simulink library "NeuroModelerLibrary"  (Simulink 10.2)
settings: Solver=ode45  StartTime=0.0  StopTime=10.0  RelTol=1e-3
libraries: $bdroot x672, simulink x5, neural x2
(part 3 of 5)

== system NeuroModelerLibrary/Simple Cells/Large PresynInh  NewNeuron v0.1 ==
  In1 : Inport
  In2 : Inport  Port=2
  In3 : Inport  Port=3
  In4 : Inport  Port=4
  In5 : Inport  Port=5
  C1 : Constant  Value=100
  C2 : Constant  Value=100
  Gain1 : Gain  Gain=0.5  OutDataTypeStr=Inherit: Same as input  ParamDataTypeStr=Inherit: Same as input
  Gain2 : Gain  Gain=-1  OutDataTypeStr=Inherit: Same as input  ParamDataTypeStr=Inherit: Same as input
  Gain3 : Gain  Gain=0.5  OutDataTypeStr=Inherit: Same as input  ParamDataTypeStr=Inherit: Same as input
  Gain4 : Gain  Gain=0.5  OutDataTypeStr=Inherit: Same as input  ParamDataTypeStr=Inherit: Same as input
  LTZone v0.1 : $bdroot/Neuron Elements/LTZone v0.1  Rc=1  Cc=0.001  RR=1  IT=0.005  T=10
  Neuro Membrane{,1..5} (6 alike) : $bdroot/Neuron Elements/Neuro Membrane v0.1  ACm=0.1  ARm=1  ECm=0.1  ERm=1
  Sum2 : Sum  InputSameDT=on  SaturateOnIntegerOverflow=on  OutDataTypeStr=Inherit: Same as first input
  Sum3 : Sum  InputSameDT=on  SaturateOnIntegerOverflow=on  OutDataTypeStr=Inherit: Same as first input
  Sum7 : Sum  Inputs=++++  InputSameDT=on  SaturateOnIntegerOverflow=on  OutDataTypeStr=Inherit: Same as first input
  Synapse PresynInh v0.1 - {1..3,5} (4 alike) : $bdroot/Neuron Elements/Synapse v0.1  SecretionTC=0.001  DecompositionTC=0.1  ksi=2  gamma=1
  Synapse PresynInh v0.1 -4 : $bdroot/Neuron Elements/Synapse v0.1  SecretionTC=0.001  DecompositionTC=0.1  ksi=2  gamma=1
  Out1 : Outport  VectorParamsAs1DForOutWhenUnconnected=off
  Out2 : Outport  Port=2  VectorParamsAs1DForOutWhenUnconnected=off
  Out3 : Outport  Port=3  VectorParamsAs1DForOutWhenUnconnected=off
  wires:
  In5/1 -> Synapse PresynInh v0.1 - 5/1
  Synapse PresynInh v0.1 - 5/1 -> Neuro Membrane5/1
  In4/1 -> Synapse PresynInh v0.1 -4/1
  Synapse PresynInh v0.1 -4/1 -> Neuro Membrane2/1
  In3/1 -> Synapse PresynInh v0.1 - 3/1
  Synapse PresynInh v0.1 - 3/1 -> Neuro Membrane3/1
  Synapse PresynInh v0.1 - 2/1 -> Neuro Membrane/1
  In2/1 -> Synapse PresynInh v0.1 - 2/1
  C2/1 -> Neuro Membrane1/2, Neuro Membrane4/2, Neuro Membrane5/2, Gain2/1
  Gain2/1 -> Neuro Membrane1/4, Neuro Membrane4/4, Neuro Membrane5/4
  Neuro Membrane2/2 -> Sum7/2
  Sum7/1 -> Gain1/1
  Neuro Membrane2/1 -> Sum7/1
  C1/1 -> LTZone v0.1/2
  In1/1 -> Synapse PresynInh v0.1 - 1/1
  Synapse PresynInh v0.1 - 1/1 -> Neuro Membrane1/1
  LTZone v0.1/1 -> Neuro Membrane4/3, Out2/1, Neuro Membrane2/3
  Neuro Membrane1/1 -> Neuro Membrane/2
  Neuro Membrane1/2 -> Neuro Membrane/4
  Neuro Membrane3/1 -> Neuro Membrane2/2
  Neuro Membrane3/2 -> Neuro Membrane2/4
  Neuro Membrane/1 -> Sum2/1
  Neuro Membrane/2 -> Sum3/1
  Sum3/1 -> Gain3/1
  Sum2/1 -> Gain4/1
  Neuro Membrane5/1 -> Sum2/2
  Neuro Membrane5/2 -> Sum3/2
  Gain1/1 -> LTZone v0.1/1
  LTZone v0.1/3 -> Out1/1
  Gain3/1 -> Neuro Membrane3/4
  Gain4/1 -> Neuro Membrane3/2
  Neuro Membrane4/1 -> Sum7/3
  Neuro Membrane4/2 -> Sum7/4
  LTZone v0.1/2 -> Out3/1

== system NeuroModelerLibrary/Simple Cells/Simple Cell ==
  Stimulate : Inport
  Arresting : Inport  Port=2
  C1 : Constant
  C2 : Constant
  C3 : Constant  Value=-1
  LTZone : $bdroot/Neuron Elements/LTZone  NM=1  FB=1.7  IT=0.005  T=0.001
  Simple Membrane : $bdroot/Neuron Elements/Simple Membrane  ACm=1e-9  ARm=1e7  ECm=1e-9  ERm=1e7  ARFm=1e8  ERFm=1e8
  Sum7 : Sum  InputSameDT=on  SaturateOnIntegerOverflow=on  OutDataTypeStr=Inherit: Same as first input
  Synapse : $bdroot/Neuron Elements/Synapse  SecretionTC=0.001  DecompositionTC=0.01  UseKsi=on  ksi=2  gamma=1e8
  Synapse1 : $bdroot/Neuron Elements/Synapse  SecretionTC=0.001  DecompositionTC=0.01  UseKsi=on  ksi=2  gamma=1e8
  Out : Outport  VectorParamsAs1DForOutWhenUnconnected=off
  Visual : Outport  Port=2  VectorParamsAs1DForOutWhenUnconnected=off
  Potential : Outport  Port=3  VectorParamsAs1DForOutWhenUnconnected=off
  wires:
  LTZone/2 -> Visual/1
  LTZone/3 -> Out/1
  C1/1 -> LTZone/2
  Stimulate/1 -> Synapse/1
  Arresting/1 -> Synapse1/1
  Sum7/1 -> LTZone/1, Potential/1
  LTZone/1 -> Simple Membrane/3
  C2/1 -> Simple Membrane/2
  C3/1 -> Simple Membrane/4
  Simple Membrane/1 -> Sum7/1
  Simple Membrane/2 -> Sum7/2
  Synapse/1 -> Simple Membrane/1
  Synapse1/1 -> Simple Membrane/5

== system NeuroModelerLibrary/Simple Cells/Simple Cell - Inertial ==
  Stimulate : Inport
  Arresting : Inport  Port=2
  C1 : Constant
  C2 : Constant
  C3 : Constant  Value=-1
  LTZone : $bdroot/Neuron Elements/LTZone  NM=1  FB=1.7  IT=0.005  T=0.00001
  Simple Membrane : $bdroot/Neuron Elements/Simple Membrane  ACm=1e-9  ARm=1e7  ECm=1e-9  ERm=1e7  ARFm=1e8  ERFm=1e8
  Simple Membrane1 : $bdroot/Neuron Elements/Simple Membrane  ACm=1e-7  ARm=1e7  ECm=1e-7  ERm=1e7  ARFm=1e8  ERFm=1e8
  Sum1 : Sum  InputSameDT=on  SaturateOnIntegerOverflow=on  OutDataTypeStr=Inherit: Same as first input
  Sum7 : Sum  InputSameDT=on  SaturateOnIntegerOverflow=on  OutDataTypeStr=Inherit: Same as first input
  Synapse : Subsystem  AncestorBlock=NeuroModelerLibrary/Neuron Elements/Synapse  mask{SecretionTC=0.001, DecompositionTC=0.01, ksi=2, gamma=1e8}
      mask prompts: SecretionTC "Mediator Secretion"; DecompositionTC "Mediator Decomposition"
  Synapse1 : Subsystem  AncestorBlock=NeuroModelerLibrary/Neuron Elements/Synapse  mask{SecretionTC=0.001, DecompositionTC=0.01, ksi=2, gamma=1e8}
      mask prompts: SecretionTC "Mediator Secretion"; DecompositionTC "Mediator Decomposition"
  Out : Outport  VectorParamsAs1DForOutWhenUnconnected=off
  Visual : Outport  Port=2  VectorParamsAs1DForOutWhenUnconnected=off
  Potential : Outport  Port=3  VectorParamsAs1DForOutWhenUnconnected=off
  wires:
  Synapse1/1(Out1) -> Simple Membrane/5
  Synapse/1(Out1) -> Simple Membrane/1
  C3/1 -> Simple Membrane/4
  C2/1 -> Simple Membrane/2
  Sum7/1 -> LTZone/1
  Arresting/1 -> Synapse1/1(In1)
  Stimulate/1 -> Synapse/1(In1)
  C1/1 -> LTZone/2
  LTZone/3 -> Out/1
  LTZone/2 -> Visual/1
  Simple Membrane/1 -> Simple Membrane1/2, Sum1/1
  Simple Membrane/2 -> Simple Membrane1/4, Sum1/2
  Simple Membrane1/1 -> Sum7/1
  Simple Membrane1/2 -> Sum7/2
  LTZone/1 -> Simple Membrane1/3
  Sum1/1 -> Potential/1

== system NeuroModelerLibrary/Simple Cells/Simple Cell MembraneCap ==
  Stimulate : Inport
  Arresting : Inport  Port=2
  C1 : Constant
  C2 : Constant
  C3 : Constant  Value=-1
  LTZone : $bdroot/Neuron Elements/LTZone  NM=1  FB=1.7  IT=0.005  T=0.00001
  Simple Membrane : $bdroot/Neuron Elements/Simple Membrane  ACm=1e-9  ARm=1e7  ECm=1e-9  ERm=1e7  ARFm=1e8  ERFm=1e8
  Simple Membrane1 : $bdroot/Neuron Elements/Simple Membrane  ACm=1e-7  ARm=1e7  ECm=1e-7  ERm=1e7  ARFm=1e8  ERFm=1e8
  Sum1 : Sum  InputSameDT=on  SaturateOnIntegerOverflow=on  OutDataTypeStr=Inherit: Same as first input
  Sum7 : Sum  InputSameDT=on  SaturateOnIntegerOverflow=on  OutDataTypeStr=Inherit: Same as first input
  Synapse : Subsystem  AncestorBlock=NeuroModelerLibrary/Neuron Elements/Synapse  mask{SecretionTC=0.001, DecompositionTC=0.01, ksi=2, gamma=1e8}
      mask prompts: SecretionTC "Mediator Secretion"; DecompositionTC "Mediator Decomposition"
  Synapse1 : Subsystem  AncestorBlock=NeuroModelerLibrary/Neuron Elements/Synapse  mask{SecretionTC=0.001, DecompositionTC=0.01, ksi=2, gamma=1e8}
      mask prompts: SecretionTC "Mediator Secretion"; DecompositionTC "Mediator Decomposition"
  Out : Outport
  Visual : Outport  Port=2
  Potential : Outport  Port=3
  wires:
  Sum1/1 -> Potential/1
  LTZone/1 -> Simple Membrane1/3
  Simple Membrane1/2 -> Sum7/2
  Simple Membrane1/1 -> Sum7/1
  Simple Membrane/2 -> Sum1/2, Simple Membrane1/4
  Simple Membrane/1 -> Sum1/1, Simple Membrane1/2
  LTZone/2 -> Visual/1
  LTZone/3 -> Out/1
  C1/1 -> LTZone/2
  Stimulate/1 -> Synapse/1(In1)
  Arresting/1 -> Synapse1/1(In1)
  Sum7/1 -> LTZone/1
  C2/1 -> Simple Membrane/2
  C3/1 -> Simple Membrane/4
  Synapse/1(Out1) -> Simple Membrane/1
  Synapse1/1(Out1) -> Simple Membrane/5

== system NeuroModelerLibrary/Simple Cells/Simple Cell MembraneCap[2] ==
  Stimulate : Inport
  Arresting : Inport  Port=2
  C1 : Constant
  C2 : Constant
  C3 : Constant  Value=-1
  LTZone : $bdroot/Neuron Elements/LTZone  NM=1  FB=1.7  IT=0.005  T=0.00001
  Scope : Scope  NumInputPorts=5
  Simple Membrane : $bdroot/Neuron Elements/Simple Membrane  ACm=1e-7  ARm=1e7  ECm=1e-7  ERm=1e7  ARFm=1e8  ERFm=1e8
  Simple Membrane1 : $bdroot/Neuron Elements/Simple Membrane  ACm=1e-7  ARm=1e7  ECm=1e-7  ERm=1e7  ARFm=1e8  ERFm=1e8
  Sum1 : Sum  InputSameDT=on  SaturateOnIntegerOverflow=on  OutDataTypeStr=Inherit: Same as first input
  Sum7 : Sum  InputSameDT=on  SaturateOnIntegerOverflow=on  OutDataTypeStr=Inherit: Same as first input
  Synapse : Subsystem  AncestorBlock=NeuroModelerLibrary/Neuron Elements/Synapse  mask{SecretionTC=0.001, DecompositionTC=0.01, ksi=2, gamma=1e8}
      mask prompts: SecretionTC "Mediator Secretion"; DecompositionTC "Mediator Decomposition"
  Synapse1 : Subsystem  AncestorBlock=NeuroModelerLibrary/Neuron Elements/Synapse  mask{SecretionTC=0.001, DecompositionTC=0.01, ksi=2, gamma=1e8}
      mask prompts: SecretionTC "Mediator Secretion"; DecompositionTC "Mediator Decomposition"
  Out : Outport
  Visual : Outport  Port=2
  Potential : Outport  Port=3
  wires:
  Sum1/1 -> Scope/2, Potential/1
  LTZone/1 -> Simple Membrane1/3
  Simple Membrane1/2 -> Sum7/2
  Simple Membrane1/1 -> Sum7/1
  Simple Membrane/2 -> Sum1/2, Simple Membrane1/4
  Simple Membrane/1 -> Sum1/1, Simple Membrane1/2
  LTZone/2 -> Visual/1
  LTZone/3 -> Out/1
  C1/1 -> LTZone/2
  Stimulate/1 -> Synapse/1(In1)
  Arresting/1 -> Synapse1/1(In1)
  Sum7/1 -> Scope/1, LTZone/1
  C2/1 -> Simple Membrane/2
  C3/1 -> Simple Membrane/4
  Synapse/1(Out1) -> Simple Membrane/1
  Synapse1/1(Out1) -> Simple Membrane/5

== system NeuroModelerLibrary/Simple Cells/Small  NewNeuron v0.1 ==
  In1 : Inport
  In2 : Inport  Port=2
  In3 : Inport  Port=3
  In4 : Inport  Port=4
  In5 : Inport  Port=5
  C1 : Constant  Value=100
  C2 : Constant  Value=100
  Gain1 : Gain  OutDataTypeStr=Inherit: Same as input  ParamDataTypeStr=Inherit: Same as input
  Gain2 : Gain  Gain=-1  OutDataTypeStr=Inherit: Same as input  ParamDataTypeStr=Inherit: Same as input
  Gain3 : Gain  Gain=0.5  OutDataTypeStr=Inherit: Same as input  ParamDataTypeStr=Inherit: Same as input
  Gain4 : Gain  Gain=0.5  OutDataTypeStr=Inherit: Same as input  ParamDataTypeStr=Inherit: Same as input
  LTZone v0.1 : $bdroot/Neuron Elements/LTZone v0.1  Rc=1  Cc=0.001  RR=1  IT=0.005  T=10
  Neuro Membrane{,1..3,5} (5 alike) : $bdroot/Neuron Elements/Neuro Membrane v0.1  ACm=0.1  ARm=1  ECm=0.1  ERm=1
  Sum2 : Sum  InputSameDT=on  SaturateOnIntegerOverflow=on  OutDataTypeStr=Inherit: Same as first input
  Sum3 : Sum  InputSameDT=on  SaturateOnIntegerOverflow=on  OutDataTypeStr=Inherit: Same as first input
  Sum7 : Sum  Inputs=++++  InputSameDT=on  SaturateOnIntegerOverflow=on  OutDataTypeStr=Inherit: Same as first input
  Synapse{1..5} (5 alike) : $bdroot/Neuron Elements/Synapse v0.1  SecretionTC=0.001  DecompositionTC=0.1  ksi=1  gamma=1
  Out1 : Outport  VectorParamsAs1DForOutWhenUnconnected=off
  Out2 : Outport  Port=2  VectorParamsAs1DForOutWhenUnconnected=off
  Out3 : Outport  Port=3  VectorParamsAs1DForOutWhenUnconnected=off
  wires:
  Gain4/1 -> Neuro Membrane3/2
  Gain3/1 -> Neuro Membrane3/4
  LTZone v0.1/3 -> Out1/1
  Gain1/1 -> LTZone v0.1/1
  Neuro Membrane5/2 -> Sum3/2
  Neuro Membrane5/1 -> Sum2/2
  Sum2/1 -> Gain4/1
  Sum3/1 -> Gain3/1
  Neuro Membrane/2 -> Sum3/1
  Neuro Membrane/1 -> Sum2/1
  Neuro Membrane3/2 -> Neuro Membrane2/4
  Neuro Membrane3/1 -> Neuro Membrane2/2
  Neuro Membrane1/2 -> Neuro Membrane/4
  Neuro Membrane1/1 -> Neuro Membrane/2
  LTZone v0.1/1 -> Neuro Membrane2/3, Out2/1
  Synapse1/1 -> Neuro Membrane1/1
  In1/1 -> Synapse1/1
  C1/1 -> LTZone v0.1/2
  Neuro Membrane2/1 -> Sum7/1
  Sum7/1 -> Gain1/1
  Neuro Membrane2/2 -> Sum7/2
  Gain2/1 -> Neuro Membrane5/4, Neuro Membrane1/4
  C2/1 -> Gain2/1, Neuro Membrane5/2, Neuro Membrane1/2
  Synapse2/1 -> Neuro Membrane/1
  In2/1 -> Synapse2/1
  Synapse3/1 -> Neuro Membrane3/1
  In3/1 -> Synapse3/1
  Synapse4/1 -> Neuro Membrane2/1
  In4/1 -> Synapse4/1
  Synapse5/1 -> Neuro Membrane5/1
  In5/1 -> Synapse5/1
  LTZone v0.1/2 -> Out3/1

== system NeuroModelerLibrary/Simple Cells/Small PresynInh NewNeuron v0.1 ==
  In1 : Inport
  In2 : Inport  Port=2
  In3 : Inport  Port=3
  In4 : Inport  Port=4
  In5 : Inport  Port=5
  C1 : Constant  Value=100
  C2 : Constant  Value=100
  Gain1 : Gain  OutDataTypeStr=Inherit: Same as input  ParamDataTypeStr=Inherit: Same as input
  Gain2 : Gain  Gain=-1  OutDataTypeStr=Inherit: Same as input  ParamDataTypeStr=Inherit: Same as input
  Gain3 : Gain  Gain=0.5  OutDataTypeStr=Inherit: Same as input  ParamDataTypeStr=Inherit: Same as input
  Gain4 : Gain  Gain=0.5  OutDataTypeStr=Inherit: Same as input  ParamDataTypeStr=Inherit: Same as input
  LTZone v0.1 : $bdroot/Neuron Elements/LTZone v0.1  Rc=1  Cc=0.001  RR=1  IT=0.005  T=10
  Neuro Membrane{,1..3,5} (5 alike) : $bdroot/Neuron Elements/Neuro Membrane v0.1  ACm=0.1  ARm=1  ECm=0.1  ERm=1
  Sum2 : Sum  InputSameDT=on  SaturateOnIntegerOverflow=on  OutDataTypeStr=Inherit: Same as first input
  Sum3 : Sum  InputSameDT=on  SaturateOnIntegerOverflow=on  OutDataTypeStr=Inherit: Same as first input
  Sum7 : Sum  Inputs=++++  InputSameDT=on  SaturateOnIntegerOverflow=on  OutDataTypeStr=Inherit: Same as first input
  Synapse PresynInh v0.1 - {1,3..5} (4 alike) : $bdroot/Neuron Elements/Synapse v0.1  SecretionTC=0.001  DecompositionTC=0.1  ksi=2  gamma=1
  "Synapse PresynInh v0.1 - 2 " : $bdroot/Neuron Elements/Synapse v0.1  SecretionTC=0.001  DecompositionTC=0.1  ksi=2  gamma=1
  Out1 : Outport  VectorParamsAs1DForOutWhenUnconnected=off
  Out2 : Outport  Port=2  VectorParamsAs1DForOutWhenUnconnected=off
  Out3 : Outport  Port=3  VectorParamsAs1DForOutWhenUnconnected=off
  wires:
  In5/1 -> Synapse PresynInh v0.1 - 5/1
  Synapse PresynInh v0.1 - 5/1 -> Neuro Membrane5/1
  In4/1 -> Synapse PresynInh v0.1 - 4/1
  Synapse PresynInh v0.1 - 4/1 -> Neuro Membrane2/1
  In3/1 -> Synapse PresynInh v0.1 - 3/1
  Synapse PresynInh v0.1 - 3/1 -> Neuro Membrane3/1
  In2/1 -> "Synapse PresynInh v0.1 - 2 "/1
  "Synapse PresynInh v0.1 - 2 "/1 -> Neuro Membrane/1
  C2/1 -> Neuro Membrane1/2, Neuro Membrane5/2, Gain2/1
  Gain2/1 -> Neuro Membrane1/4, Neuro Membrane5/4
  Neuro Membrane2/2 -> Sum7/2
  Sum7/1 -> Gain1/1
  Neuro Membrane2/1 -> Sum7/1
  C1/1 -> LTZone v0.1/2
  In1/1 -> Synapse PresynInh v0.1 - 1/1
  Synapse PresynInh v0.1 - 1/1 -> Neuro Membrane1/1
  LTZone v0.1/1 -> Out2/1, Neuro Membrane2/3
  Neuro Membrane1/1 -> Neuro Membrane/2
  Neuro Membrane1/2 -> Neuro Membrane/4
  Neuro Membrane3/1 -> Neuro Membrane2/2
  Neuro Membrane3/2 -> Neuro Membrane2/4
  Neuro Membrane/1 -> Sum2/1
  Neuro Membrane/2 -> Sum3/1
  Sum3/1 -> Gain3/1
  Sum2/1 -> Gain4/1
  Neuro Membrane5/1 -> Sum2/2
  Neuro Membrane5/2 -> Sum3/2
  Gain1/1 -> LTZone v0.1/1
  LTZone v0.1/3 -> Out1/1
  Gain3/1 -> Neuro Membrane3/4
  Gain4/1 -> Neuro Membrane3/2
  LTZone v0.1/2 -> Out3/1

== system NeuroModelerLibrary/Sized Cells/CSNM1x0 ==
  Stimulate : Inport
  Arresting : Inport  Port=2
  C1 : Constant
  C2 : Constant  Value=0.93
  C3 : Constant  Value=-1
  CSNM LTZone : $bdroot/Neuron Elements/CSNM LTZone  NM=1  FB=2  T=-0.055  switchOff=-0.1
  CSNM Synapse : $bdroot/Neuron Elements/CSNM Synapse  SecretionTC=0.001  DecompositionTC=0.005  UseKsi=off  Rs=2e7  ksi=1  U0=-0.070  Weight=1  sign=off
  CSNM Synapse1 : $bdroot/Neuron Elements/CSNM Synapse  SecretionTC=0.001  DecompositionTC=0.005  UseKsi=off  Rs=2e7  ksi=1  U0=-0.070  Weight=1  sign=off
  Simple Membrane2 : $bdroot/Neuron Elements/CSNM Compartment  ACm=1e-9  ARm=1e7  ECm=1e-9  ERm=1e7  ARFm=1e7  ERFm=1e7  U0=-0.070  sign=-1
  Sum7 : Sum  InputSameDT=on  SaturateOnIntegerOverflow=on  OutDataTypeStr=Inherit: Same as first input
  Out : Outport  VectorParamsAs1DForOutWhenUnconnected=off
  Visual : Outport  Port=2  VectorParamsAs1DForOutWhenUnconnected=off
  Potential : Outport  Port=3  VectorParamsAs1DForOutWhenUnconnected=off
  wires:
  CSNM Synapse1/1 -> Simple Membrane2/5
  Arresting/1 -> CSNM Synapse1/1
  Stimulate/1 -> CSNM Synapse/1
  CSNM Synapse/1 -> Simple Membrane2/1
  CSNM LTZone/4 -> Visual/1
  CSNM LTZone/1 -> Out/1
  C1/1 -> CSNM LTZone/2
  C2/1 -> Simple Membrane2/2
  C3/1 -> Simple Membrane2/4
  Sum7/1 -> CSNM LTZone/1
  CSNM LTZone/3 -> Simple Membrane2/3
  Simple Membrane2/1 -> Sum7/1
  Simple Membrane2/2 -> Sum7/2
  CSNM LTZone/2 -> Potential/1

== system NeuroModelerLibrary/Sized Cells/CSNM1x1 ==
  Stimulate2 : Inport
  Stimulate1 : Inport  Port=2
  Arresting1 : Inport  Port=3
  Arresting2 : Inport  Port=4
  C1 : Constant
  C2 : Constant  Value=0.93
  C3 : Constant  Value=-1
  CSNM Compartment : $bdroot/Neuron Elements/CSNM Compartment  ACm=1e-9  ARm=1e7  ECm=1e-9  ERm=1e7  ARFm=1e7  ERFm=1e7  U0=-0.070  sign=-1
  CSNM Compartment1 : $bdroot/Neuron Elements/CSNM Compartment  ACm=1e-9  ARm=1e7  ECm=1e-9  ERm=1e7  ARFm=1e7  ERFm=1e7  U0=-0.070  sign=-1
  CSNM LTZone : $bdroot/Neuron Elements/CSNM LTZone  NM=1  FB=2  T=-0.055  switchOff=-0.1
  CSNM Synapse{,1..3} (4 alike) : $bdroot/Neuron Elements/CSNM Synapse  SecretionTC=0.001  DecompositionTC=0.005  UseKsi=off  Rs=2e7  ksi=1  U0=-0.070  Weight=1  sign=off
  Sum7 : Sum  InputSameDT=on  SaturateOnIntegerOverflow=on  OutDataTypeStr=Inherit: Same as first input
  Out : Outport  VectorParamsAs1DForOutWhenUnconnected=off
  Visual : Outport  Port=2  VectorParamsAs1DForOutWhenUnconnected=off
  Potential : Outport  Port=3  VectorParamsAs1DForOutWhenUnconnected=off
  wires:
  CSNM Synapse3/1 -> CSNM Compartment/5
  Arresting2/1 -> CSNM Synapse3/1
  CSNM Synapse2/1 -> CSNM Compartment1/5
  Arresting1/1 -> CSNM Synapse2/1
  Stimulate1/1 -> CSNM Synapse/1
  CSNM Synapse/1 -> CSNM Compartment/1
  Stimulate2/1 -> CSNM Synapse1/1
  CSNM Synapse1/1 -> CSNM Compartment1/1
  C3/1 -> CSNM Compartment1/4
  C2/1 -> CSNM Compartment1/2
  CSNM LTZone/4 -> Visual/1
  CSNM LTZone/1 -> Out/1
  C1/1 -> CSNM LTZone/2
  CSNM Compartment1/1 -> CSNM Compartment/2
  CSNM Compartment1/2 -> CSNM Compartment/4
  Sum7/1 -> CSNM LTZone/1
  CSNM LTZone/3 -> CSNM Compartment/3
  CSNM Compartment/1 -> Sum7/1
  CSNM Compartment/2 -> Sum7/2
  CSNM LTZone/2 -> Potential/1

== system NeuroModelerLibrary/Sized Cells/CSNM1x2 ==
  Stimulate3 : Inport
  Stimulate2 : Inport  Port=2
  Stimulate1 : Inport  Port=3
  Arresting3 : Inport  Port=4
  Arresting2 : Inport  Port=5
  Arresting1 : Inport  Port=6
  C1 : Constant
  C2 : Constant  Value=0.93
  C3 : Constant  Value=-1
  CSNM Compartment : $bdroot/Neuron Elements/CSNM Compartment  ACm=1e-9  ARm=1e7  ECm=1e-9  ERm=1e7  ARFm=1e7  ERFm=1e7  U0=-0.070  sign=-1
  CSNM Compartment1 : $bdroot/Neuron Elements/CSNM Compartment  ACm=1e-9  ARm=1e7  ECm=1e-9  ERm=1e7  ARFm=1e7  ERFm=1e7  U0=-0.070  sign=-1
  CSNM Compartment2 : $bdroot/Neuron Elements/CSNM Compartment  ACm=1e-9  ARm=1e7  ECm=1e-9  ERm=1e7  ARFm=1e7  ERFm=1e7  U0=-0.070  sign=-1
  CSNM LTZone : $bdroot/Neuron Elements/CSNM LTZone  NM=1  FB=2  T=-0.055  switchOff=-0.1
  CSNM Synapse{,1..5} (6 alike) : $bdroot/Neuron Elements/CSNM Synapse  SecretionTC=0.001  DecompositionTC=0.005  UseKsi=off  Rs=2e7  ksi=1  U0=-0.070  Weight=1  sign=off
  Sum12 : Sum  InputSameDT=on  SaturateOnIntegerOverflow=on  OutDataTypeStr=Inherit: Same as first input
  Sum7 : Sum  InputSameDT=on  SaturateOnIntegerOverflow=on  OutDataTypeStr=Inherit: Same as first input
  Out : Outport  VectorParamsAs1DForOutWhenUnconnected=off
  Visual : Outport  Port=2  VectorParamsAs1DForOutWhenUnconnected=off
  Potential : Outport  Port=3  VectorParamsAs1DForOutWhenUnconnected=off
  wires:
  CSNM Synapse5/1 -> CSNM Compartment/5
  Arresting1/1 -> CSNM Synapse5/1
  CSNM Synapse4/1 -> CSNM Compartment1/5
  Arresting2/1 -> CSNM Synapse4/1
  CSNM Synapse3/1 -> CSNM Compartment2/5
  Arresting3/1 -> CSNM Synapse3/1
  Stimulate1/1 -> CSNM Synapse/1
  CSNM Synapse/1 -> CSNM Compartment/1
  Stimulate2/1 -> CSNM Synapse1/1
  CSNM Synapse1/1 -> CSNM Compartment1/1
  Stimulate3/1 -> CSNM Synapse2/1
  CSNM Synapse2/1 -> CSNM Compartment2/1
  C3/1 -> CSNM Compartment2/4
  C2/1 -> CSNM Compartment2/2
  CSNM Compartment2/2 -> CSNM Compartment1/4
  CSNM Compartment2/1 -> CSNM Compartment1/2
  CSNM LTZone/4 -> Visual/1
  CSNM LTZone/1 -> Out/1
  C1/1 -> CSNM LTZone/2
  CSNM Compartment1/1 -> CSNM Compartment/2, Sum12/1
  CSNM Compartment1/2 -> CSNM Compartment/4, Sum12/2
  Sum7/1 -> CSNM LTZone/1
  CSNM LTZone/3 -> CSNM Compartment/3
  CSNM Compartment/1 -> Sum7/1
  CSNM Compartment/2 -> Sum7/2
  CSNM LTZone/2 -> Potential/1

== system NeuroModelerLibrary/Sized Cells/CSNM1x3 ==
  Stimulate1 : Inport
  Stimulate2 : Inport  Port=2
  Stimulate3 : Inport  Port=3
  Stimulate4 : Inport  Port=4
  Arresting1 : Inport  Port=5
  Arresting2 : Inport  Port=6
  Arresting3 : Inport  Port=7
  Arresting4 : Inport  Port=8
  C1 : Constant
  C2 : Constant  Value=0.93
  C3 : Constant  Value=-1
  CSNM Compartment{,1..3} (4 alike) : $bdroot/Neuron Elements/CSNM Compartment  ACm=1e-9  ARm=1e7  ECm=1e-9  ERm=1e7  ARFm=1e7  ERFm=1e7  U0=-0.070  sign=-1
  CSNM LTZone : $bdroot/Neuron Elements/CSNM LTZone  NM=1  FB=2  T=-0.055  switchOff=-0.1
  CSNM Synapse{,1..7} (8 alike) : $bdroot/Neuron Elements/CSNM Synapse  SecretionTC=0.001  DecompositionTC=0.005  UseKsi=off  Rs=2e7  ksi=1  U0=-0.070  Weight=1  sign=off
  Sum12 : Sum  InputSameDT=on  SaturateOnIntegerOverflow=on  OutDataTypeStr=Inherit: Same as first input
  Sum7 : Sum  InputSameDT=on  SaturateOnIntegerOverflow=on  OutDataTypeStr=Inherit: Same as first input
  Out : Outport  VectorParamsAs1DForOutWhenUnconnected=off
  Visual : Outport  Port=2  VectorParamsAs1DForOutWhenUnconnected=off
  Potential : Outport  Port=3  VectorParamsAs1DForOutWhenUnconnected=off
  wires:
  CSNM Synapse7/1 -> CSNM Compartment/5
  Arresting4/1 -> CSNM Synapse7/1
  CSNM Synapse6/1 -> CSNM Compartment1/5
  Arresting3/1 -> CSNM Synapse6/1
  CSNM Synapse5/1 -> CSNM Compartment2/5
  Arresting2/1 -> CSNM Synapse5/1
  Stimulate4/1 -> CSNM Synapse/1
  CSNM Synapse/1 -> CSNM Compartment/1
  Stimulate3/1 -> CSNM Synapse1/1
  CSNM Synapse1/1 -> CSNM Compartment1/1
  Stimulate2/1 -> CSNM Synapse2/1
  CSNM Synapse2/1 -> CSNM Compartment2/1
  CSNM Synapse3/1 -> CSNM Compartment3/1
  C2/1 -> CSNM Compartment3/2
  C3/1 -> CSNM Compartment3/4
  CSNM Synapse4/1 -> CSNM Compartment3/5
  CSNM Compartment3/2 -> CSNM Compartment2/4
  CSNM Compartment3/1 -> CSNM Compartment2/2
  CSNM Compartment2/2 -> CSNM Compartment1/4
  CSNM Compartment2/1 -> CSNM Compartment1/2
  CSNM LTZone/4 -> Visual/1
  CSNM LTZone/1 -> Out/1
  C1/1 -> CSNM LTZone/2
  Stimulate1/1 -> CSNM Synapse3/1
  Arresting1/1 -> CSNM Synapse4/1
  CSNM Compartment1/1 -> CSNM Compartment/2, Sum12/1
  CSNM Compartment1/2 -> CSNM Compartment/4, Sum12/2
  Sum7/1 -> CSNM LTZone/1
  CSNM LTZone/3 -> CSNM Compartment/3
  CSNM Compartment/1 -> Sum7/1
  CSNM Compartment/2 -> Sum7/2
  CSNM LTZone/2 -> Potential/1

== system NeuroModelerLibrary/Sized Cells/CSNM1x4-Syn4 ==
  Stimulate1 : Inport
  Stimulate2 : Inport  Port=2
  Stimulate3 : Inport  Port=3
  Stimulate4 : Inport  Port=4
  Arresting1 : Inport  Port=5
  Arresting2 : Inport  Port=6
  Arresting3 : Inport  Port=7
  Arresting4 : Inport  Port=8
  C1 : Constant
  C2 : Constant  Value=0.93
  C3 : Constant  Value=-1
  CSNM Compartment{,1..3} (4 alike) : $bdroot/Neuron Elements/CSNM Compartment  ACm=1e-9  ARm=1e7  ECm=1e-9  ERm=1e7  ARFm=1e7  ERFm=1e7  U0=-0.070  sign=-1
  CSNM LTZone : $bdroot/Neuron Elements/CSNM LTZone  NM=1  FB=2  T=-0.055  switchOff=-0.1
  CSNM Synapse{,1..7} (8 alike) : $bdroot/Neuron Elements/CSNM Synapse  SecretionTC=0.001  DecompositionTC=0.005  UseKsi=off  Rs=2e7  ksi=1  U0=-0.070  Weight=1  sign=off
  Sum1 : Sum  Inputs=++++  InputSameDT=on  SaturateOnIntegerOverflow=on  OutDataTypeStr=Inherit: Same as first input
  Sum12 : Sum  Inputs=++++  InputSameDT=on  SaturateOnIntegerOverflow=on  OutDataTypeStr=Inherit: Same as first input
  Sum7 : Sum  InputSameDT=on  SaturateOnIntegerOverflow=on  OutDataTypeStr=Inherit: Same as first input
  Out : Outport  VectorParamsAs1DForOutWhenUnconnected=off
  Visual : Outport  Port=2  VectorParamsAs1DForOutWhenUnconnected=off
  Potential : Outport  Port=3  VectorParamsAs1DForOutWhenUnconnected=off
  wires:
  CSNM Synapse7/1 -> Sum1/4
  Arresting4/1 -> CSNM Synapse7/1
  CSNM Synapse6/1 -> Sum1/3
  Arresting3/1 -> CSNM Synapse6/1
  CSNM Synapse5/1 -> Sum1/2
  Arresting2/1 -> CSNM Synapse5/1
  Stimulate4/1 -> CSNM Synapse/1
  CSNM Synapse/1 -> Sum12/1
  Stimulate3/1 -> CSNM Synapse1/1
  CSNM Synapse1/1 -> Sum12/2
  Stimulate2/1 -> CSNM Synapse2/1
  CSNM Synapse2/1 -> Sum12/3
  CSNM Synapse3/1 -> Sum12/4
  C2/1 -> CSNM Compartment3/2
  C3/1 -> CSNM Compartment3/4
  CSNM Synapse4/1 -> Sum1/1
  CSNM Compartment3/2 -> CSNM Compartment2/4
  CSNM Compartment3/1 -> CSNM Compartment2/2
  CSNM Compartment2/2 -> CSNM Compartment1/4
  CSNM Compartment2/1 -> CSNM Compartment1/2
  CSNM LTZone/4 -> Visual/1
  CSNM LTZone/1 -> Out/1
  C1/1 -> CSNM LTZone/2
  Stimulate1/1 -> CSNM Synapse3/1
  Arresting1/1 -> CSNM Synapse4/1
  CSNM Compartment1/1 -> CSNM Compartment/2
  CSNM Compartment1/2 -> CSNM Compartment/4
  Sum7/1 -> CSNM LTZone/1
  CSNM LTZone/3 -> CSNM Compartment/3
  CSNM Compartment/1 -> Sum7/1
  CSNM Compartment/2 -> Sum7/2
  CSNM LTZone/2 -> Potential/1
  Sum1/1 -> CSNM Compartment3/5
  Sum12/1 -> CSNM Compartment3/1

== system NeuroModelerLibrary/Sized Cells/CSNM2x0 ==
  Stimulate : Inport
  Arresting : Inport  Port=2
  C1 : Constant
  C2 : Constant  Value=0.93
  C3 : Constant  Value=-1
  CSNM Compartment : $bdroot/Neuron Elements/CSNM Compartment  ACm=1e-9  ARm=1e7  ECm=1e-9  ERm=1e7  ARFm=1e7  ERFm=1e7  U0=-0.070  sign=-1
  CSNM Compartment1 : $bdroot/Neuron Elements/CSNM Compartment  ACm=1e-9  ARm=1e7  ECm=1e-9  ERm=1e7  ARFm=1e7  ERFm=1e7  U0=-0.070  sign=-1
  CSNM LTZone : $bdroot/Neuron Elements/CSNM LTZone  NM=1  FB=2  T=-0.055  switchOff=-0.1
  CSNM Synapse : $bdroot/Neuron Elements/CSNM Synapse  SecretionTC=0.001  DecompositionTC=0.005  UseKsi=off  Rs=2e7  ksi=1  U0=-0.070  Weight=1  sign=off
  CSNM Synapse1 : $bdroot/Neuron Elements/CSNM Synapse  SecretionTC=0.001  DecompositionTC=0.005  UseKsi=off  Rs=2e7  ksi=1  U0=-0.070  Weight=1  sign=off
  Sum7 : Sum  Inputs=++++  InputSameDT=on  SaturateOnIntegerOverflow=on  OutDataTypeStr=Inherit: Same as first input
  Out : Outport  VectorParamsAs1DForOutWhenUnconnected=off
  Visual : Outport  Port=2  VectorParamsAs1DForOutWhenUnconnected=off
  Potential : Outport  Port=3  VectorParamsAs1DForOutWhenUnconnected=off
  wires:
  CSNM Synapse1/1 -> CSNM Compartment/5
  Arresting/1 -> CSNM Synapse1/1
  Stimulate/1 -> CSNM Synapse/1
  CSNM Synapse/1 -> CSNM Compartment/1
  CSNM LTZone/4 -> Visual/1
  CSNM LTZone/1 -> Out/1
  C1/1 -> CSNM LTZone/2
  C2/1 -> CSNM Compartment1/2, CSNM Compartment/2
  C3/1 -> CSNM Compartment1/4, CSNM Compartment/4
  Sum7/1 -> CSNM LTZone/1
  CSNM LTZone/3 -> CSNM Compartment1/3, CSNM Compartment/3
  CSNM Compartment/1 -> Sum7/1
  CSNM Compartment/2 -> Sum7/2
  CSNM LTZone/2 -> Potential/1
  CSNM Compartment1/1 -> Sum7/3
  CSNM Compartment1/2 -> Sum7/4

== system NeuroModelerLibrary/Sized Cells/CSNM2x1 ==
  Stimulate2 : Inport
  Stimulate1 : Inport  Port=2
  Arresting1 : Inport  Port=3
  Arresting2 : Inport  Port=4
  C1 : Constant
  C2 : Constant  Value=0.93
  C3 : Constant  Value=-1
  CSNM Compartment : $bdroot/Neuron Elements/CSNM Compartment  ACm=1e-9  ARm=1e7  ECm=1e-9  ERm=1e7  ARFm=1e7  ERFm=1e7  U0=-0.070  sign=-1
  CSNM Compartment1 : $bdroot/Neuron Elements/CSNM Compartment  ACm=1e-9  ARm=1e7  ECm=1e-9  ERm=1e7  ARFm=1e7  ERFm=1e7  U0=-0.070  sign=-1
  CSNM Compartment2 : $bdroot/Neuron Elements/CSNM Compartment  ACm=1e-9  ARm=1e7  ECm=1e-9  ERm=1e7  ARFm=1e7  ERFm=1e7  U0=-0.070  sign=-1
  CSNM LTZone : $bdroot/Neuron Elements/CSNM LTZone  NM=1  FB=2  T=-0.055  switchOff=-0.1
  CSNM Synapse{,1..3} (4 alike) : $bdroot/Neuron Elements/CSNM Synapse  SecretionTC=0.001  DecompositionTC=0.005  UseKsi=off  Rs=2e7  ksi=1  U0=-0.070  Weight=1  sign=off
  Sum7 : Sum  Inputs=++++  InputSameDT=on  SaturateOnIntegerOverflow=on  OutDataTypeStr=Inherit: Same as first input
  Out : Outport  VectorParamsAs1DForOutWhenUnconnected=off
  Visual : Outport  Port=2  VectorParamsAs1DForOutWhenUnconnected=off
  Potential : Outport  Port=3  VectorParamsAs1DForOutWhenUnconnected=off
  wires:
  CSNM Synapse3/1 -> CSNM Compartment/5
  Arresting2/1 -> CSNM Synapse3/1
  CSNM Synapse2/1 -> CSNM Compartment2/5
  Arresting1/1 -> CSNM Synapse2/1
  Stimulate1/1 -> CSNM Synapse/1
  CSNM Synapse/1 -> CSNM Compartment/1
  Stimulate2/1 -> CSNM Synapse1/1
  CSNM Synapse1/1 -> CSNM Compartment2/1
  CSNM LTZone/4 -> Visual/1
  CSNM LTZone/1 -> Out/1
  C1/1 -> CSNM LTZone/2
  C2/1 -> CSNM Compartment1/2, CSNM Compartment2/2
  C3/1 -> CSNM Compartment1/4, CSNM Compartment2/4
  Sum7/1 -> CSNM LTZone/1
  CSNM LTZone/3 -> CSNM Compartment1/3, CSNM Compartment/3
  CSNM Compartment/1 -> Sum7/1
  CSNM Compartment/2 -> Sum7/2
  CSNM LTZone/2 -> Potential/1
  CSNM Compartment1/1 -> Sum7/3
  CSNM Compartment1/2 -> Sum7/4
  CSNM Compartment2/2 -> CSNM Compartment/4
  CSNM Compartment2/1 -> CSNM Compartment/2

== system NeuroModelerLibrary/Sized Cells/CSNM2x2 ==
  Stimulate3 : Inport
  Stimulate2 : Inport  Port=2
  Stimulate1 : Inport  Port=3
  Arresting3 : Inport  Port=4
  Arresting2 : Inport  Port=5
  Arresting1 : Inport  Port=6
  C1 : Constant
  C2 : Constant  Value=0.93
  C3 : Constant  Value=-1
  CSNM Compartment{,1..3} (4 alike) : $bdroot/Neuron Elements/CSNM Compartment  ACm=1e-9  ARm=1e7  ECm=1e-9  ERm=1e7  ARFm=1e7  ERFm=1e7  U0=-0.070  sign=-1
  CSNM LTZone : $bdroot/Neuron Elements/CSNM LTZone  NM=1  FB=2  T=-0.055  switchOff=-0.1
  CSNM Synapse{,1..5} (6 alike) : $bdroot/Neuron Elements/CSNM Synapse  SecretionTC=0.001  DecompositionTC=0.005  UseKsi=off  Rs=2e7  ksi=1  U0=-0.070  Weight=1  sign=off
  Sum7 : Sum  Inputs=++++  InputSameDT=on  SaturateOnIntegerOverflow=on  OutDataTypeStr=Inherit: Same as first input
  Out : Outport  VectorParamsAs1DForOutWhenUnconnected=off
  Visual : Outport  Port=2  VectorParamsAs1DForOutWhenUnconnected=off
  Potential : Outport  Port=3  VectorParamsAs1DForOutWhenUnconnected=off
  wires:
  CSNM Synapse5/1 -> CSNM Compartment/5
  Arresting1/1 -> CSNM Synapse5/1
  CSNM Synapse4/1 -> CSNM Compartment2/5
  Arresting2/1 -> CSNM Synapse4/1
  CSNM Synapse3/1 -> CSNM Compartment3/5
  Arresting3/1 -> CSNM Synapse3/1
  Stimulate1/1 -> CSNM Synapse/1
  CSNM Synapse/1 -> CSNM Compartment/1
  Stimulate2/1 -> CSNM Synapse1/1
  CSNM Synapse1/1 -> CSNM Compartment2/1
  Stimulate3/1 -> CSNM Synapse2/1
  CSNM Synapse2/1 -> CSNM Compartment3/1
  CSNM Compartment3/2 -> CSNM Compartment2/4
  CSNM Compartment3/1 -> CSNM Compartment2/2
  CSNM LTZone/4 -> Visual/1
  CSNM LTZone/1 -> Out/1
  C1/1 -> CSNM LTZone/2
  C2/1 -> CSNM Compartment3/2, CSNM Compartment1/2
  C3/1 -> CSNM Compartment3/4, CSNM Compartment1/4
  Sum7/1 -> CSNM LTZone/1
  CSNM LTZone/3 -> CSNM Compartment1/3, CSNM Compartment/3
  CSNM Compartment/1 -> Sum7/1
  CSNM Compartment/2 -> Sum7/2
  CSNM LTZone/2 -> Potential/1
  CSNM Compartment1/1 -> Sum7/3
  CSNM Compartment1/2 -> Sum7/4
  CSNM Compartment2/2 -> CSNM Compartment/4
  CSNM Compartment2/1 -> CSNM Compartment/2

== system NeuroModelerLibrary/Sized Cells/CSNM2x3 ==
  Stimulate1 : Inport
  Stimulate2 : Inport  Port=2
  Stimulate3 : Inport  Port=3
  Stimulate4 : Inport  Port=4
  Arresting1 : Inport  Port=5
  Arresting2 : Inport  Port=6
  Arresting3 : Inport  Port=7
  Arresting4 : Inport  Port=8
  C1 : Constant
  C2 : Constant  Value=0.93
  C3 : Constant  Value=-1
  CSNM Compartment{,1..4} (5 alike) : $bdroot/Neuron Elements/CSNM Compartment  ACm=1e-9  ARm=1e7  ECm=1e-9  ERm=1e7  ARFm=1e7  ERFm=1e7  U0=-0.070  sign=-1
  CSNM LTZone : $bdroot/Neuron Elements/CSNM LTZone  NM=1  FB=2  T=-0.055  switchOff=-0.1
  CSNM Synapse{,1..7} (8 alike) : $bdroot/Neuron Elements/CSNM Synapse  SecretionTC=0.001  DecompositionTC=0.005  UseKsi=off  Rs=2e7  ksi=1  U0=-0.070  Weight=1  sign=off
  Sum7 : Sum  Inputs=++++  InputSameDT=on  SaturateOnIntegerOverflow=on  OutDataTypeStr=Inherit: Same as first input
  Out : Outport  VectorParamsAs1DForOutWhenUnconnected=off
  Visual : Outport  Port=2  VectorParamsAs1DForOutWhenUnconnected=off
  Potential : Outport  Port=3  VectorParamsAs1DForOutWhenUnconnected=off
  wires:
  CSNM Synapse7/1 -> CSNM Compartment/5
  Arresting4/1 -> CSNM Synapse7/1
  CSNM Synapse6/1 -> CSNM Compartment2/5
  Arresting3/1 -> CSNM Synapse6/1
  CSNM Synapse5/1 -> CSNM Compartment3/5
  Arresting2/1 -> CSNM Synapse5/1
  Stimulate4/1 -> CSNM Synapse/1
  CSNM Synapse/1 -> CSNM Compartment/1
  Stimulate3/1 -> CSNM Synapse1/1
  CSNM Synapse1/1 -> CSNM Compartment2/1
  Stimulate2/1 -> CSNM Synapse2/1
  CSNM Synapse2/1 -> CSNM Compartment3/1
  CSNM Synapse3/1 -> CSNM Compartment4/1
  CSNM Synapse4/1 -> CSNM Compartment4/5
  CSNM Compartment4/2 -> CSNM Compartment3/4
  CSNM Compartment4/1 -> CSNM Compartment3/2
  CSNM Compartment3/2 -> CSNM Compartment2/4
  CSNM Compartment3/1 -> CSNM Compartment2/2
  CSNM LTZone/4 -> Visual/1
  CSNM LTZone/1 -> Out/1
  C1/1 -> CSNM LTZone/2
  Stimulate1/1 -> CSNM Synapse3/1
  Arresting1/1 -> CSNM Synapse4/1
  C2/1 -> CSNM Compartment1/2, CSNM Compartment4/2
  C3/1 -> CSNM Compartment1/4, CSNM Compartment4/4
  Sum7/1 -> CSNM LTZone/1
  CSNM LTZone/3 -> CSNM Compartment1/3, CSNM Compartment/3
  CSNM Compartment/1 -> Sum7/1
  CSNM Compartment/2 -> Sum7/2
  CSNM LTZone/2 -> Potential/1
  CSNM Compartment1/1 -> Sum7/3
  CSNM Compartment1/2 -> Sum7/4
  CSNM Compartment2/2 -> CSNM Compartment/4
  CSNM Compartment2/1 -> CSNM Compartment/2

== system NeuroModelerLibrary/Sized Cells/CSNM3x0 ==
  Stimulate : Inport
  Arresting : Inport  Port=2
  C1 : Constant
  C2 : Constant  Value=0.93
  C3 : Constant  Value=-1
  CSNM Compartment : $bdroot/Neuron Elements/CSNM Compartment  ACm=1e-9  ARm=1e7  ECm=1e-9  ERm=1e7  ARFm=1e7  ERFm=1e7  U0=-0.070  sign=-1
  CSNM Compartment1 : $bdroot/Neuron Elements/CSNM Compartment  ACm=1e-9  ARm=1e7  ECm=1e-9  ERm=1e7  ARFm=1e7  ERFm=1e7  U0=-0.070  sign=-1
  CSNM Compartment2 : $bdroot/Neuron Elements/CSNM Compartment  ACm=1e-9  ARm=1e7  ECm=1e-9  ERm=1e7  ARFm=1e7  ERFm=1e7  U0=-0.070  sign=-1
  CSNM LTZone : $bdroot/Neuron Elements/CSNM LTZone  NM=1  FB=2  T=-0.055  switchOff=-0.1
  CSNM Synapse : $bdroot/Neuron Elements/CSNM Synapse  SecretionTC=0.001  DecompositionTC=0.005  UseKsi=off  Rs=2e7  ksi=1  U0=-0.070  Weight=1  sign=off
  CSNM Synapse1 : $bdroot/Neuron Elements/CSNM Synapse  SecretionTC=0.001  DecompositionTC=0.005  UseKsi=off  Rs=2e7  ksi=1  U0=-0.070  Weight=1  sign=off
  Sum7 : Sum  Inputs=++++++  InputSameDT=on  SaturateOnIntegerOverflow=on  OutDataTypeStr=Inherit: Same as first input
  Out : Outport  VectorParamsAs1DForOutWhenUnconnected=off
  Visual : Outport  Port=2  VectorParamsAs1DForOutWhenUnconnected=off
  Potential : Outport  Port=3  VectorParamsAs1DForOutWhenUnconnected=off
  wires:
  CSNM Synapse1/1 -> CSNM Compartment/5
  Arresting/1 -> CSNM Synapse1/1
  Stimulate/1 -> CSNM Synapse/1
  CSNM Synapse/1 -> CSNM Compartment/1
  CSNM LTZone/4 -> Visual/1
  CSNM LTZone/1 -> Out/1
  C1/1 -> CSNM LTZone/2
  C2/1 -> CSNM Compartment/2, CSNM Compartment2/2, CSNM Compartment1/2
  C3/1 -> CSNM Compartment/4, CSNM Compartment2/4, CSNM Compartment1/4
  Sum7/1 -> CSNM LTZone/1
  CSNM LTZone/3 -> CSNM Compartment/3, CSNM Compartment2/3, CSNM Compartment1/3
  CSNM Compartment/1 -> Sum7/1
  CSNM Compartment/2 -> Sum7/2
  CSNM LTZone/2 -> Potential/1
  CSNM Compartment1/1 -> Sum7/3
  CSNM Compartment1/2 -> Sum7/4
  CSNM Compartment2/1 -> Sum7/5
  CSNM Compartment2/2 -> Sum7/6

== system NeuroModelerLibrary/Sized Cells/CSNM3x1 ==
  Stimulate2 : Inport
  Stimulate1 : Inport  Port=2
  Arresting1 : Inport  Port=3
  Arresting2 : Inport  Port=4
  C1 : Constant
  C2 : Constant  Value=0.93
  C3 : Constant  Value=-1
  CSNM Compartment{,1..3} (4 alike) : $bdroot/Neuron Elements/CSNM Compartment  ACm=1e-9  ARm=1e7  ECm=1e-9  ERm=1e7  ARFm=1e7  ERFm=1e7  U0=-0.070  sign=-1
  CSNM LTZone : $bdroot/Neuron Elements/CSNM LTZone  NM=1  FB=2  T=-0.055  switchOff=-0.1
  CSNM Synapse{,1..3} (4 alike) : $bdroot/Neuron Elements/CSNM Synapse  SecretionTC=0.001  DecompositionTC=0.005  UseKsi=off  Rs=2e7  ksi=1  U0=-0.070  Weight=1  sign=off
  Sum7 : Sum  Inputs=++++++  InputSameDT=on  SaturateOnIntegerOverflow=on  OutDataTypeStr=Inherit: Same as first input
  Out : Outport  VectorParamsAs1DForOutWhenUnconnected=off
  Visual : Outport  Port=2  VectorParamsAs1DForOutWhenUnconnected=off
  Potential : Outport  Port=3  VectorParamsAs1DForOutWhenUnconnected=off
  wires:
  CSNM Synapse3/1 -> CSNM Compartment/5
  Arresting2/1 -> CSNM Synapse3/1
  CSNM Synapse2/1 -> CSNM Compartment3/5
  Arresting1/1 -> CSNM Synapse2/1
  Stimulate1/1 -> CSNM Synapse/1
  CSNM Synapse/1 -> CSNM Compartment/1
  Stimulate2/1 -> CSNM Synapse1/1
  CSNM Synapse1/1 -> CSNM Compartment3/1
  CSNM LTZone/4 -> Visual/1
  CSNM LTZone/1 -> Out/1
  C1/1 -> CSNM LTZone/2
  C2/1 -> CSNM Compartment3/2, CSNM Compartment2/2, CSNM Compartment1/2
  C3/1 -> CSNM Compartment2/4, CSNM Compartment1/4, CSNM Compartment3/4
  Sum7/1 -> CSNM LTZone/1
  CSNM LTZone/3 -> CSNM Compartment2/3, CSNM Compartment1/3, CSNM Compartment/3
  CSNM Compartment/1 -> Sum7/1
  CSNM Compartment/2 -> Sum7/2
  CSNM LTZone/2 -> Potential/1
  CSNM Compartment1/1 -> Sum7/3
  CSNM Compartment1/2 -> Sum7/4
  CSNM Compartment2/1 -> Sum7/5
  CSNM Compartment2/2 -> Sum7/6
  CSNM Compartment3/2 -> CSNM Compartment/4
  CSNM Compartment3/1 -> CSNM Compartment/2

== system NeuroModelerLibrary/Sized Cells/CSNM3x2 ==
  Stimulate3 : Inport
  Stimulate2 : Inport  Port=2
  Stimulate1 : Inport  Port=3
  Arresting3 : Inport  Port=4
  Arresting2 : Inport  Port=5
  Arresting1 : Inport  Port=6
  C1 : Constant
  C2 : Constant  Value=0.93
  C3 : Constant  Value=-1
  CSNM Compartment{,1..4} (5 alike) : $bdroot/Neuron Elements/CSNM Compartment  ACm=1e-9  ARm=1e7  ECm=1e-9  ERm=1e7  ARFm=1e7  ERFm=1e7  U0=-0.070  sign=-1
  CSNM LTZone : $bdroot/Neuron Elements/CSNM LTZone  NM=1  FB=2  T=-0.055  switchOff=-0.1
  CSNM Synapse{,1..5} (6 alike) : $bdroot/Neuron Elements/CSNM Synapse  SecretionTC=0.001  DecompositionTC=0.005  UseKsi=off  Rs=2e7  ksi=1  U0=-0.070  Weight=1  sign=off
  Sum7 : Sum  Inputs=++++++  InputSameDT=on  SaturateOnIntegerOverflow=on  OutDataTypeStr=Inherit: Same as first input
  Out : Outport  VectorParamsAs1DForOutWhenUnconnected=off
  Visual : Outport  Port=2  VectorParamsAs1DForOutWhenUnconnected=off
  Potential : Outport  Port=3  VectorParamsAs1DForOutWhenUnconnected=off
  wires:
  CSNM Synapse5/1 -> CSNM Compartment/5
  Arresting1/1 -> CSNM Synapse5/1
  CSNM Synapse4/1 -> CSNM Compartment3/5
  Arresting2/1 -> CSNM Synapse4/1
  CSNM Synapse3/1 -> CSNM Compartment4/5
  Arresting3/1 -> CSNM Synapse3/1
  Stimulate1/1 -> CSNM Synapse/1
  CSNM Synapse/1 -> CSNM Compartment/1
  Stimulate2/1 -> CSNM Synapse1/1
  CSNM Synapse1/1 -> CSNM Compartment3/1
  Stimulate3/1 -> CSNM Synapse2/1
  CSNM Synapse2/1 -> CSNM Compartment4/1
  CSNM Compartment4/2 -> CSNM Compartment3/4
  CSNM Compartment4/1 -> CSNM Compartment3/2
  CSNM LTZone/4 -> Visual/1
  CSNM LTZone/1 -> Out/1
  C1/1 -> CSNM LTZone/2
  C2/1 -> CSNM Compartment4/2, CSNM Compartment2/2, CSNM Compartment1/2
  C3/1 -> CSNM Compartment4/4, CSNM Compartment2/4, CSNM Compartment1/4
  Sum7/1 -> CSNM LTZone/1
  CSNM LTZone/3 -> CSNM Compartment/3, CSNM Compartment2/3, CSNM Compartment1/3
  CSNM Compartment/1 -> Sum7/1
  CSNM Compartment/2 -> Sum7/2
  CSNM LTZone/2 -> Potential/1
  CSNM Compartment1/1 -> Sum7/3
  CSNM Compartment1/2 -> Sum7/4
  CSNM Compartment2/1 -> Sum7/5
  CSNM Compartment2/2 -> Sum7/6
  CSNM Compartment3/2 -> CSNM Compartment/4
  CSNM Compartment3/1 -> CSNM Compartment/2

== system NeuroModelerLibrary/Sized Cells/CSNM3x3 ==
  Stimulate1 : Inport
  Stimulate2 : Inport  Port=2
  Stimulate3 : Inport  Port=3
  Stimulate4 : Inport  Port=4
  Arresting1 : Inport  Port=5
  Arresting2 : Inport  Port=6
  Arresting3 : Inport  Port=7
  Arresting4 : Inport  Port=8
  C1 : Constant
  C2 : Constant  Value=0.93
  C3 : Constant  Value=-1
  CSNM Compartment{,1..5} (6 alike) : $bdroot/Neuron Elements/CSNM Compartment  ACm=1e-9  ARm=1e7  ECm=1e-9  ERm=1e7  ARFm=1e7  ERFm=1e7  U0=-0.070  sign=-1
  CSNM LTZone : $bdroot/Neuron Elements/CSNM LTZone  NM=1  FB=2  T=-0.055  switchOff=-0.1
  CSNM Synapse{,1..7} (8 alike) : $bdroot/Neuron Elements/CSNM Synapse  SecretionTC=0.001  DecompositionTC=0.005  UseKsi=off  Rs=2e7  ksi=1  U0=-0.070  Weight=1  sign=off
  Sum7 : Sum  Inputs=++++++  InputSameDT=on  SaturateOnIntegerOverflow=on  OutDataTypeStr=Inherit: Same as first input
  Out : Outport  VectorParamsAs1DForOutWhenUnconnected=off
  Visual : Outport  Port=2  VectorParamsAs1DForOutWhenUnconnected=off
  Potential : Outport  Port=3  VectorParamsAs1DForOutWhenUnconnected=off
  wires:
  CSNM Synapse7/1 -> CSNM Compartment/5
  Arresting4/1 -> CSNM Synapse7/1
  CSNM Synapse6/1 -> CSNM Compartment3/5
  Arresting3/1 -> CSNM Synapse6/1
  CSNM Synapse5/1 -> CSNM Compartment4/5
  Arresting2/1 -> CSNM Synapse5/1
  Stimulate4/1 -> CSNM Synapse/1
  CSNM Synapse/1 -> CSNM Compartment/1
  Stimulate3/1 -> CSNM Synapse1/1
  CSNM Synapse1/1 -> CSNM Compartment3/1
  Stimulate2/1 -> CSNM Synapse2/1
  CSNM Synapse2/1 -> CSNM Compartment4/1
  CSNM Synapse3/1 -> CSNM Compartment5/1
  CSNM Synapse4/1 -> CSNM Compartment5/5
  CSNM Compartment5/2 -> CSNM Compartment4/4
  CSNM Compartment5/1 -> CSNM Compartment4/2
  CSNM Compartment4/2 -> CSNM Compartment3/4
  CSNM Compartment4/1 -> CSNM Compartment3/2
  CSNM LTZone/4 -> Visual/1
  CSNM LTZone/1 -> Out/1
  C1/1 -> CSNM LTZone/2
  Stimulate1/1 -> CSNM Synapse3/1
  Arresting1/1 -> CSNM Synapse4/1
  C2/1 -> CSNM Compartment2/2, CSNM Compartment1/2, CSNM Compartment5/2
  C3/1 -> CSNM Compartment5/4, CSNM Compartment2/4, CSNM Compartment1/4
  Sum7/1 -> CSNM LTZone/1
  CSNM LTZone/3 -> CSNM Compartment2/3, CSNM Compartment1/3, CSNM Compartment/3
  CSNM Compartment/1 -> Sum7/1
  CSNM Compartment/2 -> Sum7/2
  CSNM LTZone/2 -> Potential/1
  CSNM Compartment1/1 -> Sum7/3
  CSNM Compartment1/2 -> Sum7/4
  CSNM Compartment2/1 -> Sum7/5
  CSNM Compartment2/2 -> Sum7/6
  CSNM Compartment3/2 -> CSNM Compartment/4
  CSNM Compartment3/1 -> CSNM Compartment/2

== system NeuroModelerLibrary/Sized Cells/CSNM4x0 ==
  Stimulate : Inport
  Arresting : Inport  Port=2
  C1 : Constant
  C2 : Constant  Value=0.93
  C3 : Constant  Value=-1
  CSNM Compartment{,1..3} (4 alike) : $bdroot/Neuron Elements/CSNM Compartment  ACm=1e-9  ARm=1e7  ECm=1e-9  ERm=1e7  ARFm=1e7  ERFm=1e7  U0=-0.070  sign=-1
  CSNM LTZone : $bdroot/Neuron Elements/CSNM LTZone  NM=1  FB=2  T=-0.055  switchOff=-0.1
  CSNM Synapse : $bdroot/Neuron Elements/CSNM Synapse  SecretionTC=0.001  DecompositionTC=0.005  UseKsi=off  Rs=2e7  ksi=1  U0=-0.070  Weight=1  sign=off
  CSNM Synapse1 : $bdroot/Neuron Elements/CSNM Synapse  SecretionTC=0.001  DecompositionTC=0.005  UseKsi=off  Rs=2e7  ksi=1  U0=-0.070  Weight=1  sign=off
  Sum7 : Sum  Inputs=++++++++  InputSameDT=on  SaturateOnIntegerOverflow=on  OutDataTypeStr=Inherit: Same as first input
  Out : Outport  VectorParamsAs1DForOutWhenUnconnected=off
  Visual : Outport  Port=2  VectorParamsAs1DForOutWhenUnconnected=off
  Potential : Outport  Port=3  VectorParamsAs1DForOutWhenUnconnected=off
  wires:
  CSNM Synapse1/1 -> CSNM Compartment/5
  Arresting/1 -> CSNM Synapse1/1
  Stimulate/1 -> CSNM Synapse/1
  CSNM Synapse/1 -> CSNM Compartment/1
  CSNM LTZone/4 -> Visual/1
  CSNM LTZone/1 -> Out/1
  C1/1 -> CSNM LTZone/2
  C2/1 -> CSNM Compartment/2, CSNM Compartment1/2, CSNM Compartment3/2, CSNM Compartment2/2
  C3/1 -> CSNM Compartment/4, CSNM Compartment1/4, CSNM Compartment3/4, CSNM Compartment2/4
  Sum7/1 -> CSNM LTZone/1
  CSNM LTZone/3 -> CSNM Compartment/3, CSNM Compartment1/3, CSNM Compartment3/3, CSNM Compartment2/3
  CSNM Compartment/1 -> Sum7/1
  CSNM Compartment/2 -> Sum7/2
  CSNM LTZone/2 -> Potential/1
  CSNM Compartment1/1 -> Sum7/3
  CSNM Compartment1/2 -> Sum7/4
  CSNM Compartment2/1 -> Sum7/5
  CSNM Compartment2/2 -> Sum7/6
  CSNM Compartment3/1 -> Sum7/7
  CSNM Compartment3/2 -> Sum7/8

== system NeuroModelerLibrary/Sized Cells/CSNM4x1 ==
  Stimulate2 : Inport
  Stimulate1 : Inport  Port=2
  Arresting1 : Inport  Port=3
  Arresting2 : Inport  Port=4
  C1 : Constant
  C2 : Constant  Value=0.93
  C3 : Constant  Value=-1
  CSNM Compartment{,1..4} (5 alike) : $bdroot/Neuron Elements/CSNM Compartment  ACm=1e-9  ARm=1e7  ECm=1e-9  ERm=1e7  ARFm=1e7  ERFm=1e7  U0=-0.070  sign=-1
  CSNM LTZone : $bdroot/Neuron Elements/CSNM LTZone  NM=1  FB=2  T=-0.055  switchOff=-0.1
  CSNM Synapse{,1..3} (4 alike) : $bdroot/Neuron Elements/CSNM Synapse  SecretionTC=0.001  DecompositionTC=0.005  UseKsi=off  Rs=2e7  ksi=1  U0=-0.070  Weight=1  sign=off
  Sum7 : Sum  Inputs=++++++++  InputSameDT=on  SaturateOnIntegerOverflow=on  OutDataTypeStr=Inherit: Same as first input
  Out : Outport  VectorParamsAs1DForOutWhenUnconnected=off
  Visual : Outport  Port=2  VectorParamsAs1DForOutWhenUnconnected=off
  Potential : Outport  Port=3  VectorParamsAs1DForOutWhenUnconnected=off
  wires:
  CSNM Synapse3/1 -> CSNM Compartment/5
  Arresting2/1 -> CSNM Synapse3/1
  CSNM Synapse2/1 -> CSNM Compartment4/5
  Arresting1/1 -> CSNM Synapse2/1
  Stimulate1/1 -> CSNM Synapse/1
  CSNM Synapse/1 -> CSNM Compartment/1
  Stimulate2/1 -> CSNM Synapse1/1
  CSNM Synapse1/1 -> CSNM Compartment4/1
  CSNM LTZone/4 -> Visual/1
  CSNM LTZone/1 -> Out/1
  C1/1 -> CSNM LTZone/2
  C2/1 -> CSNM Compartment4/2, CSNM Compartment1/2, CSNM Compartment3/2, CSNM Compartment2/2
  C3/1 -> CSNM Compartment4/4, CSNM Compartment1/4, CSNM Compartment3/4, CSNM Compartment2/4
  Sum7/1 -> CSNM LTZone/1
  CSNM LTZone/3 -> CSNM Compartment/3, CSNM Compartment1/3, CSNM Compartment3/3, CSNM Compartment2/3
  CSNM Compartment/1 -> Sum7/1
  CSNM Compartment/2 -> Sum7/2
  CSNM LTZone/2 -> Potential/1
  CSNM Compartment1/1 -> Sum7/3
  CSNM Compartment1/2 -> Sum7/4
  CSNM Compartment2/1 -> Sum7/5
  CSNM Compartment2/2 -> Sum7/6
  CSNM Compartment3/1 -> Sum7/7
  CSNM Compartment3/2 -> Sum7/8
  CSNM Compartment4/2 -> CSNM Compartment/4
  CSNM Compartment4/1 -> CSNM Compartment/2

== system NeuroModelerLibrary/Sized Cells/CSNM4x2 ==
  Stimulate3 : Inport
  Stimulate2 : Inport  Port=2
  Stimulate1 : Inport  Port=3
  Arresting3 : Inport  Port=4
  Arresting2 : Inport  Port=5
  Arresting1 : Inport  Port=6
  C1 : Constant
  C2 : Constant  Value=0.93
  C3 : Constant  Value=-1
  CSNM Compartment{,1..5} (6 alike) : $bdroot/Neuron Elements/CSNM Compartment  ACm=1e-9  ARm=1e7  ECm=1e-9  ERm=1e7  ARFm=1e7  ERFm=1e7  U0=-0.070  sign=-1
  CSNM LTZone : $bdroot/Neuron Elements/CSNM LTZone  NM=1  FB=2  T=-0.055  switchOff=-0.1
  CSNM Synapse{,1..5} (6 alike) : $bdroot/Neuron Elements/CSNM Synapse  SecretionTC=0.001  DecompositionTC=0.005  UseKsi=off  Rs=2e7  ksi=1  U0=-0.070  Weight=1  sign=off
  Sum7 : Sum  Inputs=++++++++  InputSameDT=on  SaturateOnIntegerOverflow=on  OutDataTypeStr=Inherit: Same as first input
  Out : Outport  VectorParamsAs1DForOutWhenUnconnected=off
  Visual : Outport  Port=2  VectorParamsAs1DForOutWhenUnconnected=off
  Potential : Outport  Port=3  VectorParamsAs1DForOutWhenUnconnected=off
  wires:
  CSNM Synapse5/1 -> CSNM Compartment/5
  Arresting1/1 -> CSNM Synapse5/1
  CSNM Synapse4/1 -> CSNM Compartment4/5
  Arresting2/1 -> CSNM Synapse4/1
  CSNM Synapse3/1 -> CSNM Compartment5/5
  Arresting3/1 -> CSNM Synapse3/1
  Stimulate1/1 -> CSNM Synapse/1
  CSNM Synapse/1 -> CSNM Compartment/1
  Stimulate2/1 -> CSNM Synapse1/1
  CSNM Synapse1/1 -> CSNM Compartment4/1
  Stimulate3/1 -> CSNM Synapse2/1
  CSNM Synapse2/1 -> CSNM Compartment5/1
  CSNM Compartment5/2 -> CSNM Compartment4/4
  CSNM Compartment5/1 -> CSNM Compartment4/2
  CSNM LTZone/4 -> Visual/1
  CSNM LTZone/1 -> Out/1
  C1/1 -> CSNM LTZone/2
  C2/1 -> CSNM Compartment5/2, CSNM Compartment1/2, CSNM Compartment3/2, CSNM Compartment2/2
  C3/1 -> CSNM Compartment5/4, CSNM Compartment1/4, CSNM Compartment3/4, CSNM Compartment2/4
  Sum7/1 -> CSNM LTZone/1
  CSNM LTZone/3 -> CSNM Compartment/3, CSNM Compartment1/3, CSNM Compartment3/3, CSNM Compartment2/3
  CSNM Compartment/1 -> Sum7/1
  CSNM Compartment/2 -> Sum7/2
  CSNM LTZone/2 -> Potential/1
  CSNM Compartment1/1 -> Sum7/3
  CSNM Compartment1/2 -> Sum7/4
  CSNM Compartment2/1 -> Sum7/5
  CSNM Compartment2/2 -> Sum7/6
  CSNM Compartment3/1 -> Sum7/8
  CSNM Compartment3/2 -> Sum7/7
  CSNM Compartment4/2 -> CSNM Compartment/4
  CSNM Compartment4/1 -> CSNM Compartment/2
